simulink model "TBRe18_ECU_V7_AI"  (R2017b)
settings: Solver=FixedStepDiscrete  StartTime=0.0  StopTime=inf  FixedStep=0.0001  RelTol=1e-3
PostLoadFcn:
  | model_init();
libraries: simulink x16, simulink_extras x1
(part 3 of 4)

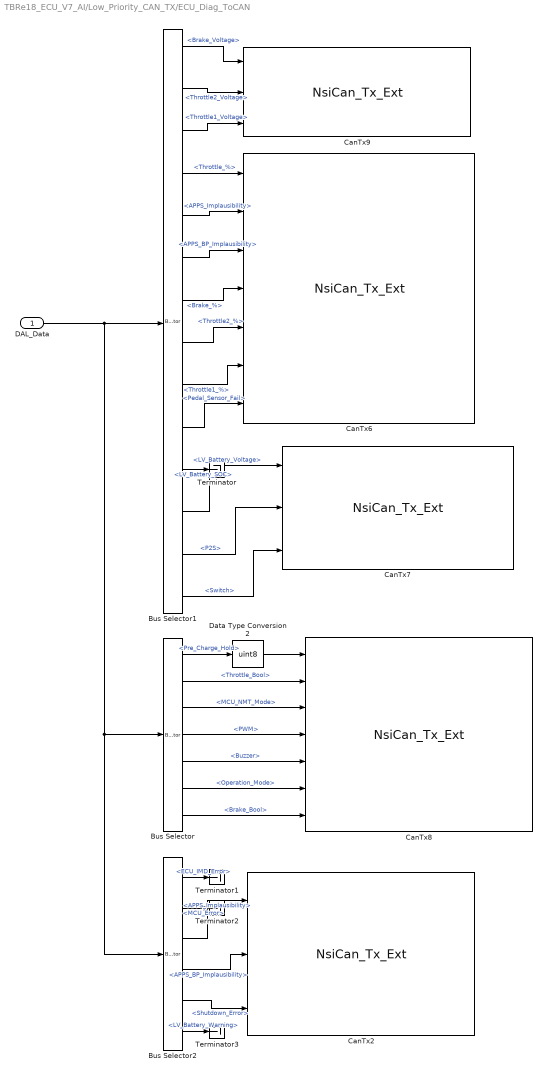
== system TBRe18_ECU_V7_AI/Low_Priority_CAN_TX/ECU_Diag_ToCAN ==
  DAL_Data : Inport
  Bus Selector : BusSelector  OutputSignals=Input_Data_Bus.BMS_Data.Pre_Charge_Hold,Vehicle_Operation_Data.Throttle_Bool,Vehicle_Operation_Data.MCU_NMT_Mode,Vehicle_Operation_Data.PWM,Vehicle_Operation_Data.Buzzer,Vehicle_Operation_Data.Operation_Mode,Vehicle_Operation_Data.Brake_Bool
  Bus Selector1 : BusSelector  OutputSignals=Input_Data_Bus.ECU_IO_Data.Pedal_Box_Data.Brake_Voltage,Input_Data_Bus.ECU_IO_Data.Pedal_Box_Data.Throttle2_Voltage,Input_Data_Bus.ECU_IO_Data.Pedal_Box_Data.Throttle1_Voltage,Input_Data_Bus.ECU_IO_Data.Pedal_Box_Data.Throttle_%,Input_Data_Bus.ECU_IO_Data.Pedal_Box_Data.APPS_Implausibility,Input_Data_Bus.ECU_IO_Data.Pedal_Box_Data.APPS_BP_Implausibility,Input_Data_Bus.ECU_IO_Data.Pedal_Box_Data.Brake_%,Input_Data_Bus.ECU_IO_Data.Pedal_Box_Data.Throttle2_%,Input_Data_Bus.ECU_IO_Data.Pedal_Box_Data.Throttle1_%,Input_Data_Bus.ECU_IO_Data.Pedal_Box_Data.Pedal_Sensor_Fail,Input_Data_Bus.ECU_IO_Data.LV_Battery_Data.LV_Battery_SOC,Input_Data_Bus.ECU_IO_Data.LV_Battery_Data.LV_Battery_Voltage,Input_Data_Bus.Console_Data.P2S,Input_Data_Bus.Console_Data.Switch
  Bus Selector2 : BusSelector  OutputSignals=Input_Data_Bus.ECU_IO_Data.IMD_Data.ECU_IMD_Error,Input_Data_Bus.MCU_Data.MCU_Error,Input_Data_Bus.ECU_IO_Data.Pedal_Box_Data.APPS_Implausibility,Input_Data_Bus.ECU_IO_Data.Pedal_Box_Data.APPS_BP_Implausibility,Input_Data_Bus.Shutdown_Data.Shutdown_Error,Input_Data_Bus.ECU_IO_Data.LV_Battery_Data.LV_Battery_Warning
  CanTx2 : S-Function  FunctionName=NsiCan_Tx_Ext  Parameters=data_can,channel,msg_name,ident,ident_type,dlc,signals,is_physical,is_canfd,is_crc  SFunctionDeploymentMode=off  EnableBusSupport=off  mask(MUXlink Can Tx){data_can=1;HIGH_SPEED;500Kbps;120 Ohm;C:\Users\TBRe-admin\Documents\MATLAB\TBRe18_DBC_190304.dbc;0;;;1;LOW_SPEED;125Kbps;560 Ohm;C:\Users\TBRe-admin\Documents\MATLAB\TBRe18_DBC_190304.dbc;0;;;0;HIGH_SPEED;1000Kbps;120 Ohm;D:\TOOLS\MUXLINK\R2011b\MUXlink\misc\BASE_CAN_MUXLAB4.dbc;0;;;0;HIGH_SPEED;500Kbps;120 Ohm;D:\TOOLS\MUXLINK\R2011b\MUXlink\misc\j1939_adapt.dbc;0;;;0;HIGH_SPEED;1000Kbps;No;D:\TOOLS\MUXLINK\R2011b\MUXlink\misc\BASE_CAN_MUXLAB4.dbc;0;;, channel=2, msg_name=ECU_Diagnostics, ident=0x700, ident_type=STD, dlc=4, signals=APPS_Implausibility;1;4;1;1.000000;0.000000;_;APPS_BP_Implausibility;1;3;1;1.000000;0.000000;_;Shutdown_Error;1;2;1;1.000000;0.000000;_, is_physical=0, is_canfd=0, is_crc=0}
      mask prompts: data_can "data can"; msg_name "msg name"
      mask help: Transmit a frame on a CAN Channel.
      mask init:
      | NsiCan_Tx_Ext_InitializationFcn();
      settings: OpenFcn=NsiCan_Tx_Ext_OpenFcn();
      mask Help:
      | eval('block=get_param(gcb, ''RTWdata'');')
      | web([docroot '\toolbox\MUXlink\html\blocks/' block.MUXlink_BlockType '.html'])
      mask Callback data_can: NsiCan_Tx_Ext_ApplyFcn(1);
      mask Callback channel: NsiCan_Tx_Ext_ApplyFcn(2);
      mask Callback msg_name: NsiCan_Tx_Ext_ApplyFcn(3);
      mask Callback ident: NsiCan_Tx_Ext_ApplyFcn(4);
      mask Callback ident_type: NsiCan_Tx_Ext_ApplyFcn(5);
      mask Callback dlc: NsiCan_Tx_Ext_ApplyFcn(6);
      mask Callback signals: NsiCan_Tx_Ext_ApplyFcn(7);
      mask Callback is_physical: NsiCan_Tx_Ext_ApplyFcn(7);
      mask Callback is_canfd: NsiCan_Tx_Ext_ApplyFcn(7);
      mask Callback is_crc: NsiCan_Tx_Ext_ApplyFcn(7);
      mask Display: image(imread('nsi.bmp'));text(0.5, 0.1, 'TX_ECU_Diagnostics_CAN2', 'horizontalAlignment', 'center', 'verticalAlignment', 'base');plot([0.05 0.05 0.05 0.05 0.05 0.05 0.05 0.05 0.05 0.05]); port_label('input',1, 'APPS_Implausibility'); port_label('input',2, 'APPS_BP_Implausibility'); port_label('input',3, 'Shutdown_Error');
  CanTx6 : S-Function  FunctionName=NsiCan_Tx_Ext  Parameters=data_can,channel,msg_name,ident,ident_type,dlc,signals,is_physical,is_canfd,is_crc  SFunctionDeploymentMode=off  EnableBusSupport=off  mask(MUXlink Can Tx){data_can=1;HIGH_SPEED;500Kbps;120 Ohm;C:\Users\TBRe-admin\Documents\MATLAB\TBRe18_DBC_190304.dbc;0;;;1;LOW_SPEED;125Kbps;560 Ohm;C:\Users\TBRe-admin\Documents\MATLAB\TBRe18_DBC_190304.dbc;0;;;0;HIGH_SPEED;1000Kbps;120 Ohm;D:\TOOLS\MUXLINK\R2011b\MUXlink\misc\BASE_CAN_MUXLAB4.dbc;0;;;0;HIGH_SPEED;500Kbps;120 Ohm;D:\TOOLS\MUXLINK\R2011b\MUXlink\misc\j1939_adapt.dbc;0;;;0;HIGH_SPEED;1000Kbps;No;D:\TOOLS\MUXLINK\R2011b\MUXlink\misc\BASE_CAN_MUXLAB4.dbc;0;;, channel=2, msg_name=ECU_Pedal_Box_Data, ident=0x702, ident_type=STD, dlc=5, signals=Throttle_Percentage;1;32;8;1.000000;0.000000;_;APPS_Implausibility;1;4;1;1.000000;0.000000;_;APPS_BP_Implausibility;1;3;1;1.000000;0.000000;_;Brake_Percentage;1;24;8;1.000000;0.000000;_;Throttle2_Percentage;1;16;8;1.000000;0.000000;_;Throttle1_Percent;1;8;8;1.000000;0.000000;_;Pedal_Sensor_Fail;1;0;3;1.000000;0.000000;_, is_physical=0, is_canfd=0, is_crc=0}
      mask prompts: data_can "data can"; msg_name "msg name"
      mask help: Transmit a frame on a CAN Channel.
      mask init:
      | NsiCan_Tx_Ext_InitializationFcn();
      settings: OpenFcn=NsiCan_Tx_Ext_OpenFcn();
      mask Help:
      | eval('block=get_param(gcb, ''RTWdata'');')
      | web([docroot '\toolbox\MUXlink\html\blocks/' block.MUXlink_BlockType '.html'])
      mask Callback data_can: NsiCan_Tx_Ext_ApplyFcn(1);
      mask Callback channel: NsiCan_Tx_Ext_ApplyFcn(2);
      mask Callback msg_name: NsiCan_Tx_Ext_ApplyFcn(3);
      mask Callback ident: NsiCan_Tx_Ext_ApplyFcn(4);
      mask Callback ident_type: NsiCan_Tx_Ext_ApplyFcn(5);
      mask Callback dlc: NsiCan_Tx_Ext_ApplyFcn(6);
      mask Callback signals: NsiCan_Tx_Ext_ApplyFcn(7);
      mask Callback is_physical: NsiCan_Tx_Ext_ApplyFcn(7);
      mask Callback is_canfd: NsiCan_Tx_Ext_ApplyFcn(7);
      mask Callback is_crc: NsiCan_Tx_Ext_ApplyFcn(7);
      mask Display: image(imread('nsi.bmp'));text(0.5, 0.1, 'TX_ECU_Pedal_Box_Data_CAN2', 'horizontalAlignment', 'center', 'verticalAlignment', 'base');plot([0.05 0.05 0.05 0.05 0.05 0.05 0.05 0.05 0.05 0.05]); port_label('input',1, 'Throttle_Percentage'); port_label('input',2, 'APPS_Implausibility'); port_label('input',3, 'APPS_BP_Implausibility'); port_label('input',4, 'Brake_Percentage'); port_label('input',5, 'Throttle2_Percentage'); port_label('input',6, 'Throttle1_Percent'); port_label('input',7, 'Pedal_Sensor_Fail');
  CanTx7 : S-Function  FunctionName=NsiCan_Tx_Ext  Parameters=data_can,channel,msg_name,ident,ident_type,dlc,signals,is_physical,is_canfd,is_crc  SFunctionDeploymentMode=off  EnableBusSupport=off  mask(MUXlink Can Tx){data_can=1;HIGH_SPEED;500Kbps;120 Ohm;C:\Users\TBRe-admin\Documents\MATLAB\TBRe18_DBC_190304.dbc;0;;;1;LOW_SPEED;125Kbps;560 Ohm;C:\Users\TBRe-admin\Documents\MATLAB\TBRe18_DBC_190304.dbc;0;;;0;HIGH_SPEED;1000Kbps;120 Ohm;D:\TOOLS\MUXLINK\R2011b\MUXlink\misc\BASE_CAN_MUXLAB4.dbc;0;;;0;HIGH_SPEED;500Kbps;120 Ohm;D:\TOOLS\MUXLINK\R2011b\MUXlink\misc\j1939_adapt.dbc;0;;;0;HIGH_SPEED;1000Kbps;No;D:\TOOLS\MUXLINK\R2011b\MUXlink\misc\BASE_CAN_MUXLAB4.dbc;0;;, channel=2, msg_name=ECU_HW_IO, ident=0x701, ident_type=STD, dlc=4, signals=LV_Battery_Voltage;1;16;16;1.000000;0.000000;mV;Console_Push_to_Start;1;9;1;1.000000;0.000000;Bool;Console_Reset;1;8;1;1.000000;0.000000;Bool, is_physical=0, is_canfd=0, is_crc=0}
      mask prompts: data_can "data can"; msg_name "msg name"
      mask help: Transmit a frame on a CAN Channel.
      mask init:
      | NsiCan_Tx_Ext_InitializationFcn();
      settings: OpenFcn=NsiCan_Tx_Ext_OpenFcn();
      mask Help:
      | eval('block=get_param(gcb, ''RTWdata'');')
      | web([docroot '\toolbox\MUXlink\html\blocks/' block.MUXlink_BlockType '.html'])
      mask Callback data_can: NsiCan_Tx_Ext_ApplyFcn(1);
      mask Callback channel: NsiCan_Tx_Ext_ApplyFcn(2);
      mask Callback msg_name: NsiCan_Tx_Ext_ApplyFcn(3);
      mask Callback ident: NsiCan_Tx_Ext_ApplyFcn(4);
      mask Callback ident_type: NsiCan_Tx_Ext_ApplyFcn(5);
      mask Callback dlc: NsiCan_Tx_Ext_ApplyFcn(6);
      mask Callback signals: NsiCan_Tx_Ext_ApplyFcn(7);
      mask Callback is_physical: NsiCan_Tx_Ext_ApplyFcn(7);
      mask Callback is_canfd: NsiCan_Tx_Ext_ApplyFcn(7);
      mask Callback is_crc: NsiCan_Tx_Ext_ApplyFcn(7);
      mask Display: image(imread('nsi.bmp'));text(0.5, 0.1, 'TX_ECU_HW_IO_CAN2', 'horizontalAlignment', 'center', 'verticalAlignment', 'base');plot([0.05 0.05 0.05 0.05 0.05 0.05 0.05 0.05 0.05 0.05]); port_label('input',1, 'LV_Battery_Voltage'); port_label('input',2, 'Console_Push_to_Start'); port_label('input',3, 'Console_Reset');
  CanTx8 : S-Function  FunctionName=NsiCan_Tx_Ext  Parameters=data_can,channel,msg_name,ident,ident_type,dlc,signals,is_physical,is_canfd,is_crc  SFunctionDeploymentMode=off  EnableBusSupport=off  mask(MUXlink Can Tx){data_can=1;HIGH_SPEED;500Kbps;120 Ohm;C:\Users\TBRe-admin\Documents\MATLAB\TBRe18_DBC_190304.dbc;0;;;1;LOW_SPEED;125Kbps;560 Ohm;C:\Users\TBRe-admin\Documents\MATLAB\TBRe18_DBC_190304.dbc;0;;;0;HIGH_SPEED;1000Kbps;120 Ohm;D:\TOOLS\MUXLINK\R2011b\MUXlink\misc\BASE_CAN_MUXLAB4.dbc;0;;;0;HIGH_SPEED;500Kbps;120 Ohm;D:\TOOLS\MUXLINK\R2011b\MUXlink\misc\j1939_adapt.dbc;0;;;0;HIGH_SPEED;1000Kbps;No;D:\TOOLS\MUXLINK\R2011b\MUXlink\misc\BASE_CAN_MUXLAB4.dbc;0;;, channel=2, msg_name=ECU_Vehicle_Functionality, ident=0x704, ident_type=STD, dlc=4, signals=Pre_Charge;1;24;8;1.000000;0.000000;_;Throttle_Bool;1;2;1;1.000000;0.000000;_;MCU_NMT_Mode;1;16;8;1.000000;0.000000;_;PWM;1;3;1;1.000000;0.000000;_;Buzzer;1;1;1;1.000000;0.000000;_;Vehicle_Operation;1;8;8;1.000000;0.000000;_;Brake_Bool;1;0;1;1.000000;0.000000;_, is_physical=0, is_canfd=0, is_crc=0}
      mask prompts: data_can "data can"; msg_name "msg name"
      mask help: Transmit a frame on a CAN Channel.
      mask init:
      | NsiCan_Tx_Ext_InitializationFcn();
      settings: OpenFcn=NsiCan_Tx_Ext_OpenFcn();
      mask Help:
      | eval('block=get_param(gcb, ''RTWdata'');')
      | web([docroot '\toolbox\MUXlink\html\blocks/' block.MUXlink_BlockType '.html'])
      mask Callback data_can: NsiCan_Tx_Ext_ApplyFcn(1);
      mask Callback channel: NsiCan_Tx_Ext_ApplyFcn(2);
      mask Callback msg_name: NsiCan_Tx_Ext_ApplyFcn(3);
      mask Callback ident: NsiCan_Tx_Ext_ApplyFcn(4);
      mask Callback ident_type: NsiCan_Tx_Ext_ApplyFcn(5);
      mask Callback dlc: NsiCan_Tx_Ext_ApplyFcn(6);
      mask Callback signals: NsiCan_Tx_Ext_ApplyFcn(7);
      mask Callback is_physical: NsiCan_Tx_Ext_ApplyFcn(7);
      mask Callback is_canfd: NsiCan_Tx_Ext_ApplyFcn(7);
      mask Callback is_crc: NsiCan_Tx_Ext_ApplyFcn(7);
      mask Display: image(imread('nsi.bmp'));text(0.5, 0.1, 'TX_ECU_Vehicle_Functionality_CAN2', 'horizontalAlignment', 'center', 'verticalAlignment', 'base');plot([0.05 0.05 0.05 0.05 0.05 0.05 0.05 0.05 0.05 0.05]); port_label('input',1, 'Pre_Charge'); port_label('input',2, 'Throttle_Bool'); port_label('input',3, 'MCU_NMT_Mode'); port_label('input',4, 'PWM'); port_label('input',5, 'Buzzer'); port_label('input',6, 'Vehicle_Operation'); port_label('input',7, 'Brake_Bool');
  CanTx9 : S-Function  FunctionName=NsiCan_Tx_Ext  Parameters=data_can,channel,msg_name,ident,ident_type,dlc,signals,is_physical,is_canfd,is_crc  SFunctionDeploymentMode=off  EnableBusSupport=off  mask(MUXlink Can Tx){data_can=1;HIGH_SPEED;500Kbps;120 Ohm;C:\Users\TBRe-admin\Documents\MATLAB\TBRe18_DBC_190304.dbc;0;;;1;LOW_SPEED;125Kbps;560 Ohm;C:\Users\TBRe-admin\Documents\MATLAB\TBRe18_DBC_190304.dbc;0;;;0;HIGH_SPEED;1000Kbps;120 Ohm;D:\TOOLS\MUXLINK\R2011b\MUXlink\misc\BASE_CAN_MUXLAB4.dbc;0;;;0;HIGH_SPEED;500Kbps;120 Ohm;D:\TOOLS\MUXLINK\R2011b\MUXlink\misc\j1939_adapt.dbc;0;;;0;HIGH_SPEED;1000Kbps;No;D:\TOOLS\MUXLINK\R2011b\MUXlink\misc\BASE_CAN_MUXLAB4.dbc;0;;, channel=2, msg_name=ECU_Pedal_Voltages, ident=0x703, ident_type=STD, dlc=8, signals=Brake_Voltage;1;32;16;1.000000;0.000000;mV;Throttle2_Voltage;1;48;16;1.000000;0.000000;_;Throttle1_Voltage;1;0;16;1.000000;0.000000;_, is_physical=0, is_canfd=0, is_crc=0}
      mask prompts: data_can "data can"; msg_name "msg name"
      mask help: Transmit a frame on a CAN Channel.
      mask init:
      | NsiCan_Tx_Ext_InitializationFcn();
      settings: OpenFcn=NsiCan_Tx_Ext_OpenFcn();
      mask Help:
      | eval('block=get_param(gcb, ''RTWdata'');')
      | web([docroot '\toolbox\MUXlink\html\blocks/' block.MUXlink_BlockType '.html'])
      mask Callback data_can: NsiCan_Tx_Ext_ApplyFcn(1);
      mask Callback channel: NsiCan_Tx_Ext_ApplyFcn(2);
      mask Callback msg_name: NsiCan_Tx_Ext_ApplyFcn(3);
      mask Callback ident: NsiCan_Tx_Ext_ApplyFcn(4);
      mask Callback ident_type: NsiCan_Tx_Ext_ApplyFcn(5);
      mask Callback dlc: NsiCan_Tx_Ext_ApplyFcn(6);
      mask Callback signals: NsiCan_Tx_Ext_ApplyFcn(7);
      mask Callback is_physical: NsiCan_Tx_Ext_ApplyFcn(7);
      mask Callback is_canfd: NsiCan_Tx_Ext_ApplyFcn(7);
      mask Callback is_crc: NsiCan_Tx_Ext_ApplyFcn(7);
      mask Display: image(imread('nsi.bmp'));text(0.5, 0.1, 'TX_ECU_Pedal_Voltages_CAN2', 'horizontalAlignment', 'center', 'verticalAlignment', 'base');plot([0.05 0.05 0.05 0.05 0.05 0.05 0.05 0.05 0.05 0.05]); port_label('input',1, 'Brake_Voltage'); port_label('input',2, 'Throttle2_Voltage'); port_label('input',3, 'Throttle1_Voltage');
  Data Type Conversion2 : DataTypeConversion  OutDataTypeStr=uint8
  Terminator{,1..3} (4 alike) : Terminator
  wires:
  Bus Selector1/4 -> CanTx6/1  "<Throttle_%>"
  Bus Selector1/5 -> CanTx6/2  "<APPS_Implausibility>"
  Bus Selector1/6 -> CanTx6/3  "<APPS_BP_Implausibility>"
  Bus Selector1/7 -> CanTx6/4  "<Brake_%>"
  Bus Selector1/8 -> CanTx6/5  "<Throttle2_%>"
  Bus Selector1/9 -> CanTx6/6  "<Throttle1_%>"
  Bus Selector1/10 -> CanTx6/7  "<Pedal_Sensor_Fail>"
  Bus Selector1/1 -> CanTx9/1  "<Brake_Voltage>"
  Bus Selector1/2 -> CanTx9/2  "<Throttle2_Voltage>"
  Bus Selector1/3 -> CanTx9/3  "<Throttle1_Voltage>"
  Bus Selector/7 -> CanTx8/7  "<Brake_Bool>"
  Bus Selector2/4 -> CanTx2/2  "<APPS_BP_Implausibility>"
  Bus Selector1/13 -> CanTx7/2  "<P2S>"
  Bus Selector/2 -> CanTx8/2  "<Throttle_Bool>"
  Bus Selector/3 -> CanTx8/3  "<MCU_NMT_Mode>"
  Bus Selector/4 -> CanTx8/4  "<PWM>"
  Bus Selector/6 -> CanTx8/6  "<Operation_Mode>"
  Bus Selector/5 -> CanTx8/5  "<Buzzer>"
  DAL_Data/1 -> Bus Selector1/1, Bus Selector/1, Bus Selector2/1
  Bus Selector2/5 -> CanTx2/3  "<Shutdown_Error>"
  Bus Selector2/3 -> CanTx2/1  "<APPS_Implausibility>"
  Data Type Conversion2/1 -> CanTx8/1
  Bus Selector/1 -> Data Type Conversion2/1  "<Pre_Charge_Hold>"
  Bus Selector1/12 -> CanTx7/1  "<LV_Battery_Voltage>"
  Bus Selector1/14 -> CanTx7/3  "<Switch>"
  Bus Selector1/11 -> Terminator/1  "<LV_Battery_SOC>"
  Bus Selector2/1 -> Terminator1/1  "<ECU_IMD_Error>"
  Bus Selector2/2 -> Terminator2/1  "<MCU_Error>"
  Bus Selector2/6 -> Terminator3/1  "<LV_Battery_Warning>"

== system TBRe18_ECU_V7_AI/Low_Priority_CAN_TX/Init ==

== system TBRe18_ECU_V7_AI/Low_Priority_CAN_TX/MCU_Diag_ToCAN ==
  DAL_Data : Inport
  Bus Selector : BusSelector  OutputSignals=Input_Data_Bus.MCU_Data.DC_Link_Current,Input_Data_Bus.MCU_Data.DC_Link_Voltage,Input_Data_Bus.MCU_Data.Motor_Temp,Input_Data_Bus.MCU_Data.MCU_Temp
  CanRx1 : S-Function  FunctionName=NsiCan_Rx_Ext  Parameters=data_can,channel,msg_name,ident,ident_type,dlc,signals,is_trigger,is_physical,is_canfd,is_rxgw  SFunctionDeploymentMode=off  EnableBusSupport=off  mask(MUXlink Can Rx){data_can=1;HIGH_SPEED;500Kbps;120 Ohm;C:\Users\TBRe-admin\Documents\MATLAB\TBRe18_DBC_190304.dbc;0;;;1;LOW_SPEED;125Kbps;560 Ohm;C:\Users\TBRe-admin\Documents\MATLAB\TBRe18_DBC_190304.dbc;0;;;0;HIGH_SPEED;1000Kbps;120 Ohm;D:\TOOLS\MUXLINK\R2011b\MUXlink\misc\BASE_CAN_MUXLAB4.dbc;0;;;0;HIGH_SPEED;500Kbps;120 Ohm;D:\TOOLS\MUXLINK\R2011b\MUXlink\misc\j1939_adapt.dbc;0;;;0;HIGH_SPEED;1000Kbps;No;D:\TOOLS\MUXLINK\R2011b\MUXlink\misc\BASE_CAN_MUXLAB4.dbc;0;;, channel=1, msg_name=MCU_TPDO3, ident=0x381, ident_type=STD, dlc=8, signals=MCU_Error_Code;1;0;-16;1.000000;0.000000;_;MCU_Status_Word;1;16;16;1.000000;0.000000;_;MCU_PhaseB_Current;1;48;-16;1.000000;0.000000;_;MCU_PhaseA_Current;1;32;-16;1.000000;0.000000;_, is_trigger=0, is_physical=0, is_canfd=0, is_rxgw=0}
      mask prompts: data_can "data can"; msg_name "msg name"
      mask help: Receive a frame from a CAN channel.
      mask init:
      | NsiCan_Rx_Ext_InitializationFcn();
      settings: OpenFcn=NsiCan_Rx_Ext_OpenFcn();
      mask Help:
      | eval('block=get_param(gcb, ''RTWdata'');')
      | web([docroot '\toolbox\MUXlink\html\blocks/' block.MUXlink_BlockType '.html'])
      mask Callback data_can: NsiCan_Rx_Ext_ApplyFcn(1);
      mask Callback channel: NsiCan_Rx_Ext_ApplyFcn(2);
      mask Callback msg_name: NsiCan_Rx_Ext_ApplyFcn(3);
      mask Callback ident: NsiCan_Rx_Ext_ApplyFcn(4);
      mask Callback ident_type: NsiCan_Rx_Ext_ApplyFcn(5);
      mask Callback dlc: NsiCan_Rx_Ext_ApplyFcn(6);
      mask Callback signals: NsiCan_Rx_Ext_ApplyFcn(7);
      mask Callback is_trigger: NsiCan_Rx_Ext_ApplyFcn(8);
      mask Callback is_physical: NsiCan_Rx_Ext_ApplyFcn(9);
      mask Callback is_canfd: NsiCan_Rx_Ext_ApplyFcn(10);
      mask Callback is_rxgw: NsiCan_Rx_Ext_ApplyFcn(11);
      mask Display: image(imread('nsi.bmp'));text(0.5, 0.3, 'RX_MCU_TPDO3_CAN1', 'horizontalAlignment', 'center', 'verticalAlignment', 'base');plot([0.05 0.05 0.05 0.05 0.05 0.05 0.05 0.05 0.05 0.05]); port_label('output',1, 'MCU_Error_Code'); port_label('output',2, 'MCU_Status_Word'); port_label('output',3, 'MCU_PhaseB_Current'); port_label('output',4, 'MCU_PhaseA_Current'); port_label('output',5, 'Status');
  CanRx2 : S-Function  FunctionName=NsiCan_Rx_Ext  Parameters=data_can,channel,msg_name,ident,ident_type,dlc,signals,is_trigger,is_physical,is_canfd,is_rxgw  SFunctionDeploymentMode=off  EnableBusSupport=off  mask(MUXlink Can Rx){data_can=1;HIGH_SPEED;500Kbps;120 Ohm;C:\Users\TBRe-admin\Documents\MATLAB\TBRe18_DBC_190304.dbc;0;;;1;LOW_SPEED;125Kbps;560 Ohm;C:\Users\TBRe-admin\Documents\MATLAB\TBRe18_DBC_190304.dbc;0;;;0;HIGH_SPEED;1000Kbps;120 Ohm;D:\TOOLS\MUXLINK\R2011b\MUXlink\misc\BASE_CAN_MUXLAB4.dbc;0;;;0;HIGH_SPEED;500Kbps;120 Ohm;D:\TOOLS\MUXLINK\R2011b\MUXlink\misc\j1939_adapt.dbc;0;;;0;HIGH_SPEED;1000Kbps;No;D:\TOOLS\MUXLINK\R2011b\MUXlink\misc\BASE_CAN_MUXLAB4.dbc;0;;, channel=1, msg_name=MCU_TPDO4, ident=0x481, ident_type=STD, dlc=8, signals=MCU_DC_Power;1;0;-32;1.000000;0.000000;W;MCU_Velocity_Actual_Value;1;32;-32;1.000000;0.000000;_, is_trigger=0, is_physical=0, is_canfd=0, is_rxgw=0}
      mask prompts: data_can "data can"; msg_name "msg name"
      mask help: Receive a frame from a CAN channel.
      mask init:
      | NsiCan_Rx_Ext_InitializationFcn();
      settings: OpenFcn=NsiCan_Rx_Ext_OpenFcn();
      mask Help:
      | eval('block=get_param(gcb, ''RTWdata'');')
      | web([docroot '\toolbox\MUXlink\html\blocks/' block.MUXlink_BlockType '.html'])
      mask Callback data_can: NsiCan_Rx_Ext_ApplyFcn(1);
      mask Callback channel: NsiCan_Rx_Ext_ApplyFcn(2);
      mask Callback msg_name: NsiCan_Rx_Ext_ApplyFcn(3);
      mask Callback ident: NsiCan_Rx_Ext_ApplyFcn(4);
      mask Callback ident_type: NsiCan_Rx_Ext_ApplyFcn(5);
      mask Callback dlc: NsiCan_Rx_Ext_ApplyFcn(6);
      mask Callback signals: NsiCan_Rx_Ext_ApplyFcn(7);
      mask Callback is_trigger: NsiCan_Rx_Ext_ApplyFcn(8);
      mask Callback is_physical: NsiCan_Rx_Ext_ApplyFcn(9);
      mask Callback is_canfd: NsiCan_Rx_Ext_ApplyFcn(10);
      mask Callback is_rxgw: NsiCan_Rx_Ext_ApplyFcn(11);
      mask Display: image(imread('nsi.bmp'));text(0.5, 0.3, 'RX_MCU_TPDO4_CAN1', 'horizontalAlignment', 'center', 'verticalAlignment', 'base');plot([0.05 0.05 0.05 0.05 0.05 0.05 0.05 0.05 0.05 0.05]); port_label('output',1, 'MCU_DC_Power'); port_label('output',2, 'MCU_Velocity_Actual_Value'); port_label('output',3, 'Status');
  CanTx2 : S-Function  FunctionName=NsiCan_Tx_Ext  Parameters=data_can,channel,msg_name,ident,ident_type,dlc,signals,is_physical,is_canfd,is_crc  SFunctionDeploymentMode=off  EnableBusSupport=off  mask(MUXlink Can Tx){data_can=1;HIGH_SPEED;500Kbps;120 Ohm;C:\Users\TBRe-admin\Documents\MATLAB\TBRe18_DBC_190304.dbc;0;;;1;LOW_SPEED;125Kbps;560 Ohm;C:\Users\TBRe-admin\Documents\MATLAB\TBRe18_DBC_190304.dbc;0;;;0;HIGH_SPEED;1000Kbps;120 Ohm;D:\TOOLS\MUXLINK\R2011b\MUXlink\misc\BASE_CAN_MUXLAB4.dbc;0;;;0;HIGH_SPEED;500Kbps;120 Ohm;D:\TOOLS\MUXLINK\R2011b\MUXlink\misc\j1939_adapt.dbc;0;;;0;HIGH_SPEED;1000Kbps;No;D:\TOOLS\MUXLINK\R2011b\MUXlink\misc\BASE_CAN_MUXLAB4.dbc;0;;, channel=1, msg_name=MCU_TPDO4, ident=0x481, ident_type=STD, dlc=8, signals=MCU_DC_Power;1;0;-32;1.000000;0.000000;W;MCU_Velocity_Actual_Value;1;32;-32;1.000000;0.000000;_, is_physical=0, is_canfd=0, is_crc=0}
      mask prompts: data_can "data can"; msg_name "msg name"
      mask help: Transmit a frame on a CAN Channel.
      mask init:
      | NsiCan_Tx_Ext_InitializationFcn();
      settings: OpenFcn=NsiCan_Tx_Ext_OpenFcn();
      mask Help:
      | eval('block=get_param(gcb, ''RTWdata'');')
      | web([docroot '\toolbox\MUXlink\html\blocks/' block.MUXlink_BlockType '.html'])
      mask Callback data_can: NsiCan_Tx_Ext_ApplyFcn(1);
      mask Callback channel: NsiCan_Tx_Ext_ApplyFcn(2);
      mask Callback msg_name: NsiCan_Tx_Ext_ApplyFcn(3);
      mask Callback ident: NsiCan_Tx_Ext_ApplyFcn(4);
      mask Callback ident_type: NsiCan_Tx_Ext_ApplyFcn(5);
      mask Callback dlc: NsiCan_Tx_Ext_ApplyFcn(6);
      mask Callback signals: NsiCan_Tx_Ext_ApplyFcn(7);
      mask Callback is_physical: NsiCan_Tx_Ext_ApplyFcn(7);
      mask Callback is_canfd: NsiCan_Tx_Ext_ApplyFcn(7);
      mask Callback is_crc: NsiCan_Tx_Ext_ApplyFcn(7);
      mask Display: image(imread('nsi.bmp'));text(0.5, 0.3, 'TX_MCU_TPDO4_CAN1', 'horizontalAlignment', 'center', 'verticalAlignment', 'base');plot([0.05 0.05 0.05 0.05 0.05 0.05 0.05 0.05 0.05 0.05]); port_label('input',1, 'MCU_DC_Power'); port_label('input',2, 'MCU_Velocity_Actual_Value');
  CanTx3 : S-Function  FunctionName=NsiCan_Tx_Ext  Parameters=data_can,channel,msg_name,ident,ident_type,dlc,signals,is_physical,is_canfd,is_crc  SFunctionDeploymentMode=off  EnableBusSupport=off  mask(MUXlink Can Tx){data_can=1;HIGH_SPEED;500Kbps;120 Ohm;C:\Users\TBRe-admin\Documents\MATLAB\TBRe18_DBC_190304.dbc;0;;;1;LOW_SPEED;125Kbps;560 Ohm;C:\Users\TBRe-admin\Documents\MATLAB\TBRe18_DBC_190304.dbc;0;;;0;HIGH_SPEED;1000Kbps;120 Ohm;D:\TOOLS\MUXLINK\R2011b\MUXlink\misc\BASE_CAN_MUXLAB4.dbc;0;;;0;HIGH_SPEED;500Kbps;120 Ohm;D:\TOOLS\MUXLINK\R2011b\MUXlink\misc\j1939_adapt.dbc;0;;;0;HIGH_SPEED;1000Kbps;No;D:\TOOLS\MUXLINK\R2011b\MUXlink\misc\BASE_CAN_MUXLAB4.dbc;0;;, channel=2, msg_name=MCU_TPDO2, ident=0x281, ident_type=STD, dlc=8, signals=MCU_DC_Link_Current;1;32;-32;1.000000;0.000000;_;MCU_DC_Link_Voltage;1;16;-16;1.000000;0.000000;_;Motor_Temp;1;8;8;1.000000;0.000000;_;MCU_Temp;1;0;8;1.000000;0.000000;_, is_physical=0, is_canfd=0, is_crc=0}
      mask prompts: data_can "data can"; msg_name "msg name"
      mask help: Transmit a frame on a CAN Channel.
      mask init:
      | NsiCan_Tx_Ext_InitializationFcn();
      settings: OpenFcn=NsiCan_Tx_Ext_OpenFcn();
      mask Help:
      | eval('block=get_param(gcb, ''RTWdata'');')
      | web([docroot '\toolbox\MUXlink\html\blocks/' block.MUXlink_BlockType '.html'])
      mask Callback data_can: NsiCan_Tx_Ext_ApplyFcn(1);
      mask Callback channel: NsiCan_Tx_Ext_ApplyFcn(2);
      mask Callback msg_name: NsiCan_Tx_Ext_ApplyFcn(3);
      mask Callback ident: NsiCan_Tx_Ext_ApplyFcn(4);
      mask Callback ident_type: NsiCan_Tx_Ext_ApplyFcn(5);
      mask Callback dlc: NsiCan_Tx_Ext_ApplyFcn(6);
      mask Callback signals: NsiCan_Tx_Ext_ApplyFcn(7);
      mask Callback is_physical: NsiCan_Tx_Ext_ApplyFcn(7);
      mask Callback is_canfd: NsiCan_Tx_Ext_ApplyFcn(7);
      mask Callback is_crc: NsiCan_Tx_Ext_ApplyFcn(7);
      mask Display: image(imread('nsi.bmp'));text(0.5, 0.3, 'TX_MCU_TPDO2_CAN2', 'horizontalAlignment', 'center', 'verticalAlignment', 'base');plot([0.05 0.05 0.05 0.05 0.05 0.05 0.05 0.05 0.05 0.05]); port_label('input',1, 'MCU_DC_Link_Current'); port_label('input',2, 'MCU_DC_Link_Voltage'); port_label('input',3, 'Motor_Temp'); port_label('input',4, 'MCU_Temp');
  CanTx4 : S-Function  FunctionName=NsiCan_Tx_Ext  Parameters=data_can,channel,msg_name,ident,ident_type,dlc,signals,is_physical,is_canfd,is_crc  SFunctionDeploymentMode=off  EnableBusSupport=off  mask(MUXlink Can Tx){data_can=1;HIGH_SPEED;500Kbps;120 Ohm;C:\Users\TBRe-admin\Documents\MATLAB\TBRe18_DBC_190304.dbc;0;;;1;LOW_SPEED;125Kbps;560 Ohm;C:\Users\TBRe-admin\Documents\MATLAB\TBRe18_DBC_190304.dbc;0;;;0;HIGH_SPEED;1000Kbps;120 Ohm;D:\TOOLS\MUXLINK\R2011b\MUXlink\misc\BASE_CAN_MUXLAB4.dbc;0;;;0;HIGH_SPEED;500Kbps;120 Ohm;D:\TOOLS\MUXLINK\R2011b\MUXlink\misc\j1939_adapt.dbc;0;;;0;HIGH_SPEED;1000Kbps;No;D:\TOOLS\MUXLINK\R2011b\MUXlink\misc\BASE_CAN_MUXLAB4.dbc;0;;, channel=1, msg_name=MCU_TPDO3, ident=0x381, ident_type=STD, dlc=8, signals=MCU_Error_Code;1;0;-16;1.000000;0.000000;_;MCU_Status_Word;1;16;16;1.000000;0.000000;_;MCU_PhaseB_Current;1;48;-16;1.000000;0.000000;_;MCU_PhaseA_Current;1;32;-16;1.000000;0.000000;_, is_physical=0, is_canfd=0, is_crc=0}
      mask prompts: data_can "data can"; msg_name "msg name"
      mask help: Transmit a frame on a CAN Channel.
      mask init:
      | NsiCan_Tx_Ext_InitializationFcn();
      settings: OpenFcn=NsiCan_Tx_Ext_OpenFcn();
      mask Help:
      | eval('block=get_param(gcb, ''RTWdata'');')
      | web([docroot '\toolbox\MUXlink\html\blocks/' block.MUXlink_BlockType '.html'])
      mask Callback data_can: NsiCan_Tx_Ext_ApplyFcn(1);
      mask Callback channel: NsiCan_Tx_Ext_ApplyFcn(2);
      mask Callback msg_name: NsiCan_Tx_Ext_ApplyFcn(3);
      mask Callback ident: NsiCan_Tx_Ext_ApplyFcn(4);
      mask Callback ident_type: NsiCan_Tx_Ext_ApplyFcn(5);
      mask Callback dlc: NsiCan_Tx_Ext_ApplyFcn(6);
      mask Callback signals: NsiCan_Tx_Ext_ApplyFcn(7);
      mask Callback is_physical: NsiCan_Tx_Ext_ApplyFcn(7);
      mask Callback is_canfd: NsiCan_Tx_Ext_ApplyFcn(7);
      mask Callback is_crc: NsiCan_Tx_Ext_ApplyFcn(7);
      mask Display: image(imread('nsi.bmp'));text(0.5, 0.3, 'TX_MCU_TPDO3_CAN1', 'horizontalAlignment', 'center', 'verticalAlignment', 'base');plot([0.05 0.05 0.05 0.05 0.05 0.05 0.05 0.05 0.05 0.05]); port_label('input',1, 'MCU_Error_Code'); port_label('input',2, 'MCU_Status_Word'); port_label('input',3, 'MCU_PhaseB_Current'); port_label('input',4, 'MCU_PhaseA_Current');
  Data Type Conversion : DataTypeConversion  OutDataTypeStr=uint16  LockScale=on
  Data Type Conversion1 : DataTypeConversion  OutDataTypeStr=uint32
  Terminator1 : Terminator
  Terminator2 : Terminator
  wires:
  CanRx2/1 -> CanTx2/1
  CanRx2/2 -> CanTx2/2
  CanRx1/1 -> CanTx4/1
  CanRx1/2 -> CanTx4/2
  CanRx1/3 -> CanTx4/3
  CanRx1/4 -> CanTx4/4
  Bus Selector/3 -> CanTx3/3  "<Motor_Temp>"
  Bus Selector/4 -> CanTx3/4  "<MCU_Temp>"
  Bus Selector/2 -> Data Type Conversion/1  "<DC_Link_Voltage>"
  CanRx1/5 -> Terminator1/1
  DAL_Data/1 -> Bus Selector/1
  Data Type Conversion/1 -> CanTx3/2
  CanRx2/3 -> Terminator2/1
  Bus Selector/1 -> Data Type Conversion1/1  "<DC_Link_Current>"
  Data Type Conversion1/1 -> CanTx3/1

== system TBRe18_ECU_V7_AI/Data_Processing/Diagnostics/BMS_Diagnostics ==
  note: SDO data is reply from MCU DC Link Voltage read request when not in ready to drive, see HP CAN out
  In1 : Inport
  Bus Creator : BusCreator  Inputs=1
  Bus Selector : BusSelector  OutputSignals=LP_CAN_RX.BMS_Data.Instant_Pack_Voltage,HP_CAN_RX.MCU_DC_Link_Voltage,HP_CAN_RX.SDO_Data
  Compare To Constant : simulink/Logic and Bit Operations/Compare To Constant  relop===  const=3.0  OutDataTypeStr=boolean
  Data Store Read : DataStoreRead  DataStoreName=O_M
  Delay : Delay  DelayLength=10  InitialCondition=0
  MATLAB Function : MATLAB Function  TreatAsAtomicUnit=on
  Switch : Switch  Criteria=u2 > Threshold
  Out1 : Outport
  wires:
  Bus Creator/1 -> Out1/1
  In1/1 -> Bus Selector/1
  Bus Selector/1 -> MATLAB Function/1(Pack_Voltage)  "<Instant_Pack_Voltage>"
  MATLAB Function/1(Pre_Charge_Hold) -> Bus Creator/1  "Pre_Charge_Hold"
  Switch/1 -> MATLAB Function/2(MCU_Link_Voltage)
  Bus Selector/2 -> Switch/1  "<MCU_DC_Link_Voltage>"
  Bus Selector/3 -> Switch/3  "<SDO_Data>"
  Data Store Read/1 -> Compare To Constant/1
  Compare To Constant/1 -> Delay/1
  Delay/1 -> Switch/2

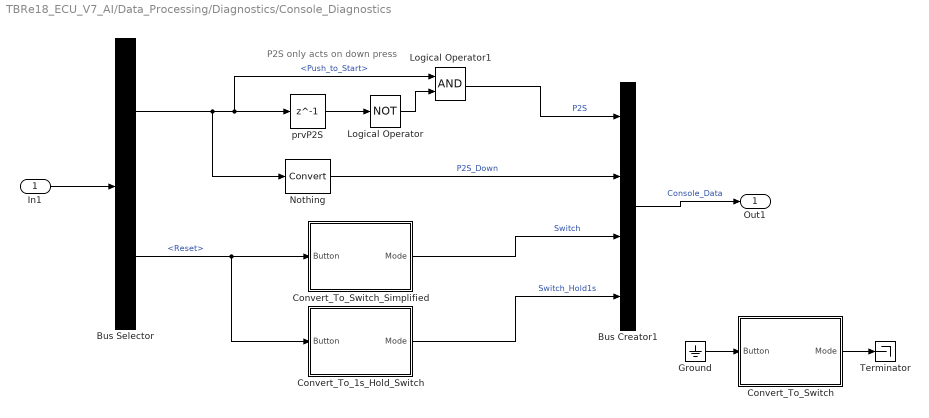
== system TBRe18_ECU_V7_AI/Data_Processing/Diagnostics/Console_Diagnostics ==
  note: P2S only acts on down press
  In1 : Inport
  Bus Creator1 : BusCreator  Inputs=4
  Bus Selector : BusSelector  OutputSignals=Hardwired_Inputs.Console_Data.Push_to_Start,Hardwired_Inputs.Console_Data.Reset
  Convert_To_1s_Hold_Switch : Subsystem  mask{initPos=false}
      mask prompts: initPos "Initial Position"
  Convert_To_Switch : Subsystem  mask{initPos=false}
      mask prompts: initPos "Initial Position"
  Convert_To_Switch_Simplified : Subsystem  mask{initPos=false}
      mask prompts: initPos "Initial Position"
  Ground : Ground
  Logical Operator : Logic  Operator=NOT  AllPortsSameDT=off  OutDataTypeStr=boolean
  Logical Operator1 : Logic  AllPortsSameDT=off  OutDataTypeStr=boolean
  Nothing : DataTypeConversion
  Terminator : Terminator
  prvP2S : Delay  DelayLength=1  InitialCondition=0
  Out1 : Outport
  wires:
  Logical Operator/1 -> Logical Operator1/2
  prvP2S/1 -> Logical Operator/1
  Logical Operator1/1 -> Bus Creator1/1  "P2S"
  Bus Creator1/1 -> Out1/1  "Console_Data"
  Bus Selector/1 -> Nothing/1, Logical Operator1/1, prvP2S/1  "<Push_to_Start>"
  Bus Selector/2 -> Convert_To_Switch_Simplified/1(Button), Convert_To_1s_Hold_Switch/1(Button)  "<Reset>"
  Convert_To_Switch_Simplified/1(Mode) -> Bus Creator1/3  "Switch"
  In1/1 -> Bus Selector/1
  Nothing/1 -> Bus Creator1/2  "P2S_Down"
  Convert_To_1s_Hold_Switch/1(Mode) -> Bus Creator1/4  "Switch_Hold1s"
  Ground/1 -> Convert_To_Switch/1(Button)
  Convert_To_Switch/1(Mode) -> Terminator/1

== system TBRe18_ECU_V7_AI/Data_Processing/Diagnostics/ECU_I//0s_Diagnostics ==
  In1 : Inport
  AIR : Subsystem
  Bus Creator : BusCreator  Inputs=4
  Bus Selector : BusSelector  OutputSignals=Hardwired_Inputs
  IMD : Subsystem
  LV_Battery : Subsystem
  Pedal_Box : Subsystem
  Out1 : Outport
  wires:
  In1/1 -> Bus Selector/1
  Bus Selector/1 -> IMD/1(In1), AIR/1(In1), LV_Battery/1(In1), Pedal_Box/1(In1)  "<Hardwired_Inputs>"
  Pedal_Box/1(Out1) -> Bus Creator/1  "Pedal_Box_Data"
  LV_Battery/1(Out1) -> Bus Creator/2  "LV_Battery_Data"
  IMD/1(Out1) -> Bus Creator/3  "IMD_Data"
  AIR/1(Out1) -> Bus Creator/4  "AIR_Data"
  Bus Creator/1 -> Out1/1

== system TBRe18_ECU_V7_AI/Data_Processing/Diagnostics/MCU_Diagnostics ==
  In1 : Inport
  Bus Creator : BusCreator  Inputs=15
  Bus Selector : BusSelector  OutputSignals=HP_CAN_RX.Motor_Temp,HP_CAN_RX.MCU_Temp
  Bus Selector1 : BusSelector  OutputSignals=HP_CAN_RX.OD_Index,HP_CAN_RX.OD_Sub_Index,HP_CAN_RX.SDO_Data
  Configuration_Check : Subsystem  Commented=on
  Error_Check : simulink/Logic and Bit Operations/Compare To Zero  Commented=on  relop=~=  OutDataTypeStr=boolean
  MCU_Error : Logic  Commented=on  Operator=OR  AllPortsSameDT=off  OutDataTypeStr=boolean
  Power Monitoring : Subsystem  Commented=on
  Temp_Check : Subsystem
  Out1 : Outport
  wires:
  Bus Creator/1 -> Out1/1
  Error_Check/1 -> MCU_Error/1
  Temp_Check/1(MCU_Temperature) -> Bus Creator/7  "MCU_Temp"
  Temp_Check/2(Motor_Temperature) -> Bus Creator/8  "Motor_Temp"
  Temp_Check/3(MCU_Motor_Temp_Error) -> Bus Creator/9  "MCU_Motor_Temp_Error"
  Temp_Check/4(MCU_Pump_Req) -> Bus Creator/10  "MCU_Pump_Req"
  MCU_Error/1 -> Bus Creator/11  "MCU_Error"
  In1/1 -> Bus Selector/1, Bus Selector1/1
  Power Monitoring/1(MCU_Power) -> Bus Creator/12  "MCU_Power"
  Power Monitoring/2(DC_Link_Voltage) -> Bus Creator/13  "DC_Link_Voltage"
  Power Monitoring/3(DC_Link_Current) -> Bus Creator/14  "DC_Link_Current"
  Power Monitoring/4(Power_Limit_Breach) -> Bus Creator/15  "Power_Limit_Breach"
  Bus Selector1/1 -> Configuration_Check/1(OD_Index_In)  "<OD_Index>"
  Bus Selector1/2 -> Configuration_Check/2(OD_Sub_Index_In)  "<OD_Sub_Index>"
  Bus Selector1/3 -> Configuration_Check/3(SDO_Data_In)  "<SDO_Data>"
  Configuration_Check/1(SDO_Specifier) -> Bus Creator/1  "SDO_Specifier"
  Configuration_Check/2(OD_Index_Out) -> Bus Creator/2  "OD_Index_Out"
  Configuration_Check/3(OD_Sub_Index_Out) -> Bus Creator/3  "OD_Sub_Index"
  Configuration_Check/4(SDO_Data_Out) -> Bus Creator/4  "SDO_Data_Out"
  Configuration_Check/5(MCU_Config_Error) -> Bus Creator/5  "MCU_Config_Error"
  Bus Selector/1 -> Temp_Check/1(MCU_Temp)  "<Motor_Temp>"
  Configuration_Check/6(MCU_Config_Parameter_No) -> Bus Creator/6  "MCU_Config_Param_No"
  Bus Selector/2 -> Temp_Check/2(Motor_Temp)  "<MCU_Temp>"

== system TBRe18_ECU_V7_AI/Data_Processing/Diagnostics/Shutdown_System_Diagnostics ==
  In1 : Inport
  Bus Creator : BusCreator  Inputs=1
  Constant : Constant  Value=false
  Terminator : Terminator
  Out1 : Outport
  wires:
  Bus Creator/1 -> Out1/1
  Constant/1 -> Bus Creator/1  "Shutdown_Error"
  In1/1 -> Terminator/1

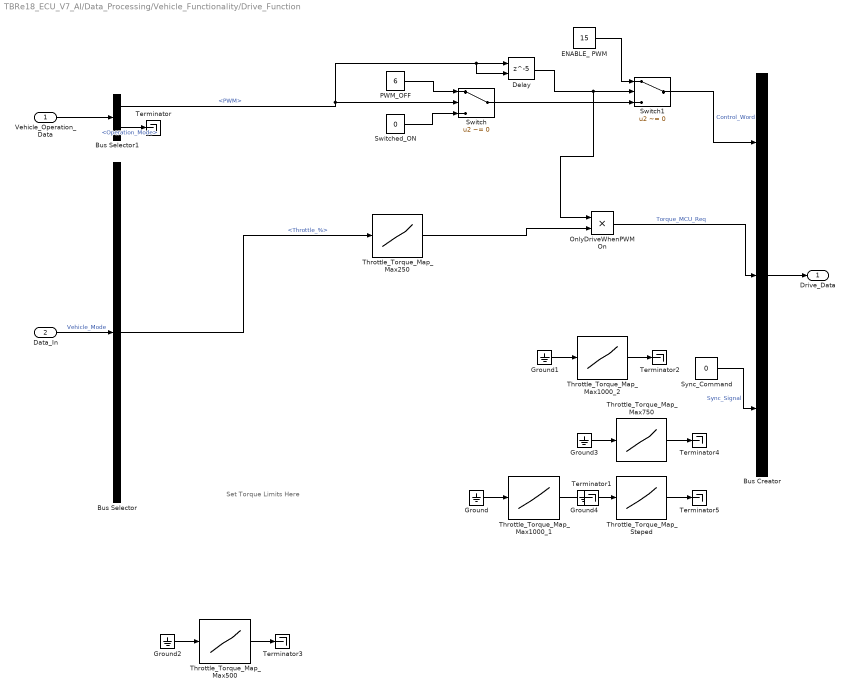
== system TBRe18_ECU_V7_AI/Data_Processing/Vehicle_Functionality/Drive_Function ==
  note: Set Torque Limits Here
  Vehicle_Operation_Data : Inport
  Data_In : Inport  Port=2
  Bus Creator : BusCreator  Inputs=3
  Bus Selector : BusSelector  OutputSignals=ECU_IO_Data.Pedal_Box_Data.Throttle_%
  Bus Selector1 : BusSelector  OutputSignals=PWM,Operation_Mode
  Delay : Delay  DelayLength=5  ExternalReset=Falling
      settings: InputPortMap=u0,r5
  ENABLE_ PWM : Constant  Value=15  OutDataTypeStr=uint16
  Ground{,1..4} (5 alike) : Ground
  OnlyDriveWhenPWMOn : Product  OutDataTypeStr=int16
  PWM_OFF : Constant  Value=6  OutDataTypeStr=uint16
  Switch : Switch  Criteria=u2 ~= 0  OutDataTypeStr=uint16
  Switch1 : Switch  Criteria=u2 ~= 0  OutDataTypeStr=uint16
  Switched_ON : Constant  Value=0  OutDataTypeStr=uint16
  "Sync_Command " : Constant  Value=0  OutDataTypeStr=uint8  SampleTime=-1
  Terminator{,1..5} (6 alike) : Terminator
  Throttle_Torque_Map_Max1000_1 : Lookup_n-D  NumberOfTableDimensions=1  BreakpointsForDimension1=[0,30,75,95,100]  Table=[0,100,650,800,1000]  ExtrapMethod=Clip  UseLastTableValue=on  InternalRulePriority=Speed  OutDataTypeStr=uint16  RndMeth=Simplest  InputSameDT=on
  Throttle_Torque_Map_Max1000_2 : Lookup_n-D  NumberOfTableDimensions=1  BreakpointsForDimension1=[0,30,75,95,100]  Table=[0,100,650,800,1000]  ExtrapMethod=Clip  UseLastTableValue=on  InternalRulePriority=Speed  OutDataTypeStr=uint16  RndMeth=Simplest  InputSameDT=on
  Throttle_Torque_Map_Max250 : Lookup_n-D  NumberOfTableDimensions=1  BreakpointsForDimension1=[0,30,75,100]  Table=[0,15,200,250]  ExtrapMethod=Clip  UseLastTableValue=on  InternalRulePriority=Speed  OutDataTypeStr=int16  RndMeth=Simplest  InputSameDT=on
  Throttle_Torque_Map_Max500 : Lookup_n-D  NumberOfTableDimensions=1  BreakpointsForDimension1=[0,30,75,100]  Table=[0,30,400,500]  ExtrapMethod=Clip  UseLastTableValue=on  InternalRulePriority=Speed  OutDataTypeStr=int16  RndMeth=Simplest  InputSameDT=on
  Throttle_Torque_Map_Max750 : Lookup_n-D  NumberOfTableDimensions=1  BreakpointsForDimension1=[0,30,75,100]  Table=[0,100,600,750]  ExtrapMethod=Clip  UseLastTableValue=on  InternalRulePriority=Speed  OutDataTypeStr=uint16  RndMeth=Simplest  InputSameDT=on
  Throttle_Torque_Map_Steped : Lookup_n-D  NumberOfTableDimensions=1  BreakpointsForDimension1=[0,20,40,60,70,90,100]  Table=[0,90,500,500,800,800,1000]  ExtrapMethod=Clip  UseLastTableValue=on  InternalRulePriority=Speed  OutDataTypeStr=uint16  RndMeth=Simplest  InputSameDT=on
  Drive_Data : Outport
  wires:
  "Sync_Command "/1 -> Bus Creator/3  "Sync_Signal"
  PWM_OFF/1 -> Switch/1
  Switched_ON/1 -> Switch/3
  Switch/1 -> Switch1/3
  ENABLE_ PWM/1 -> Switch1/1
  Delay/1 -> OnlyDriveWhenPWMOn/1, Switch1/2
  Switch1/1 -> Bus Creator/1  "Control_Word"
  Bus Creator/1 -> Drive_Data/1
  OnlyDriveWhenPWMOn/1 -> Bus Creator/2  "Torque_MCU_Req"
  Data_In/1 -> Bus Selector/1  "Vehicle_Mode"
  Vehicle_Operation_Data/1 -> Bus Selector1/1
  Bus Selector1/1 -> Delay/2, Delay/1, Switch/2  "<PWM>"
  Throttle_Torque_Map_Max250/1 -> OnlyDriveWhenPWMOn/2
  Bus Selector/1 -> Throttle_Torque_Map_Max250/1  "<Throttle_%>"
  Bus Selector1/2 -> Terminator/1  "<Operation_Mode>"
  Ground/1 -> Throttle_Torque_Map_Max1000_1/1
  Throttle_Torque_Map_Max1000_1/1 -> Terminator1/1
  Ground1/1 -> Throttle_Torque_Map_Max1000_2/1
  Throttle_Torque_Map_Max1000_2/1 -> Terminator2/1
  Ground2/1 -> Throttle_Torque_Map_Max500/1
  Throttle_Torque_Map_Max500/1 -> Terminator3/1
  Ground3/1 -> Throttle_Torque_Map_Max750/1
  Throttle_Torque_Map_Max750/1 -> Terminator4/1
  Ground4/1 -> Throttle_Torque_Map_Steped/1
  Throttle_Torque_Map_Steped/1 -> Terminator5/1

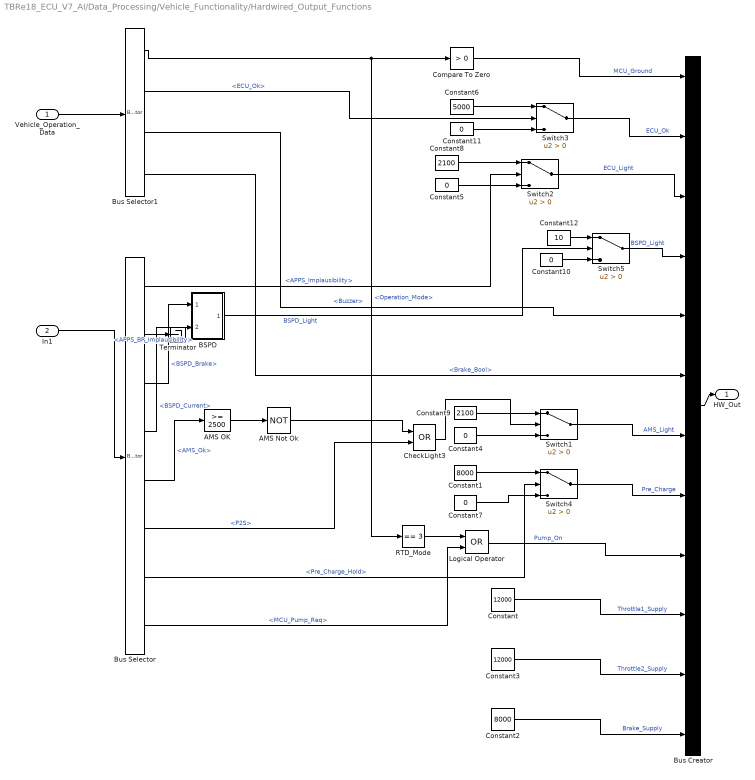
== system TBRe18_ECU_V7_AI/Data_Processing/Vehicle_Functionality/Hardwired_Output_Functions ==
  Vehicle_Operation_Data : Inport
  In1 : Inport  Port=2
  AMS Not Ok : Logic  Operator=NOT  AllPortsSameDT=off  OutDataTypeStr=boolean
  AMS OK : simulink/Logic and Bit Operations/Compare To Constant  relop=>=  const=2500  OutDataTypeStr=boolean
  BSPD : Subsystem
  Bus Creator : BusCreator  Inputs=12
  Bus Selector : BusSelector  OutputSignals=ECU_IO_Data.Pedal_Box_Data.APPS_Implausibility,ECU_IO_Data.Pedal_Box_Data.APPS_BP_Implausibility,Raw_Input_Data.Hardwired_Inputs.Pedal_Box_Data.BSPD_Brake,Raw_Input_Data.Hardwired_Inputs.Pedal_Box_Data.BSPD_Current,Raw_Input_Data.Hardwired_Inputs.AMS_Ok,Console_Data.P2S,BMS_Data.Pre_Charge_Hold,MCU_Data.MCU_Pump_Req
  Bus Selector1 : BusSelector  OutputSignals=Operation_Mode,ECU_Ok,Buzzer,Brake_Bool
  CheckLight3 : Logic  Operator=OR  AllPortsSameDT=off  OutDataTypeStr=boolean
  Compare To Zero : simulink/Logic and Bit Operations/Compare To Zero  relop=>  OutDataTypeStr=boolean
  Constant : Constant  Value=12000  OutDataTypeStr=uint16
  Constant1 : Constant  Value=8000  OutDataTypeStr=Inherit: Inherit via back propagation
  Constant{4..5,10..11} (4 alike) : Constant  Value=0  OutDataTypeStr=uint16
  Constant12 : Constant  Value=10  OutDataTypeStr=uint16
  Constant2 : Constant  Value=8000  OutDataTypeStr=uint16
  Constant3 : Constant  Value=12000  OutDataTypeStr=uint16
  Constant6 : Constant  Value=5000  OutDataTypeStr=uint16
  Constant7 : Constant  Value=0  OutDataTypeStr=Inherit: Inherit via back propagation
  Constant8 : Constant  Value=2100  OutDataTypeStr=uint16
  Constant9 : Constant  Value=2100  OutDataTypeStr=uint16
  Logical Operator : Logic  Operator=OR  AllPortsSameDT=off  OutDataTypeStr=boolean
  RTD_Mode : simulink/Logic and Bit Operations/Compare To Constant  relop===  const=3  OutDataTypeStr=boolean
  Switch1 : Switch  Criteria=u2 > Threshold  OutDataTypeStr=uint16
  Switch2 : Switch  Criteria=u2 > Threshold
  Switch3 : Switch  Criteria=u2 > Threshold
  Switch4 : Switch  Criteria=u2 > Threshold  OutDataTypeStr=uint16
  Switch5 : Switch  Criteria=u2 > Threshold
  Terminator : Terminator
  HW_Out : Outport
  wires:
  Constant/1 -> Bus Creator/10  "Throttle1_Supply"
  Bus Creator/1 -> HW_Out/1
  Constant2/1 -> Bus Creator/12  "Brake_Supply"
  Constant3/1 -> Bus Creator/11  "Throttle2_Supply"
  In1/1 -> Bus Selector/1
  Bus Selector/8 -> Logical Operator/2  "<MCU_Pump_Req>"
  Compare To Zero/1 -> Bus Creator/1  "MCU_Ground"
  Switch1/1 -> Bus Creator/7  "AMS_Light"
  Bus Selector/5 -> AMS OK/1  "<AMS_Ok>"
  Switch4/1 -> Bus Creator/8  "Pre_Charge"
  Switch3/1 -> Bus Creator/2  "ECU_Ok"
  Constant1/1 -> Switch4/1
  Bus Selector/7 -> Switch4/2  "<Pre_Charge_Hold>"
  Constant6/1 -> Switch3/1
  Constant7/1 -> Switch4/3
  Vehicle_Operation_Data/1 -> Bus Selector1/1
  Bus Selector1/1 -> Compare To Zero/1, RTD_Mode/1  "<Operation_Mode>"
  Bus Selector1/2 -> Switch3/2  "<ECU_Ok>"
  Constant4/1 -> Switch1/3
  Constant9/1 -> Switch1/1
  Constant11/1 -> Switch3/3
  Bus Selector/4 -> BSPD/2(In3)  "<BSPD_Current>"
  Bus Selector/3 -> BSPD/1(In1)  "<BSPD_Brake>"
  AMS OK/1 -> AMS Not Ok/1
  Bus Selector/6 -> CheckLight3/2  "<P2S>"
  CheckLight3/1 -> Switch1/2
  AMS Not Ok/1 -> CheckLight3/1
  Bus Selector1/4 -> Bus Creator/6  "<Brake_Bool>"
  Bus Selector1/3 -> Bus Creator/5  "<Buzzer>"
  BSPD/1(Out1) -> Switch5/2  "BSPD_Light"
  Bus Selector/1 -> Switch2/2  "<APPS_Implausibility>"
  RTD_Mode/1 -> Logical Operator/1
  Logical Operator/1 -> Bus Creator/9  "Pump_On"
  Switch2/1 -> Bus Creator/3  "ECU_Light"
  Constant5/1 -> Switch2/3
  Constant8/1 -> Switch2/1
  Switch5/1 -> Bus Creator/4  "BSPD_Light"
  Constant12/1 -> Switch5/1
  Constant10/1 -> Switch5/3
  Bus Selector/2 -> Terminator/1  "<APPS_BP_Implausibility>"

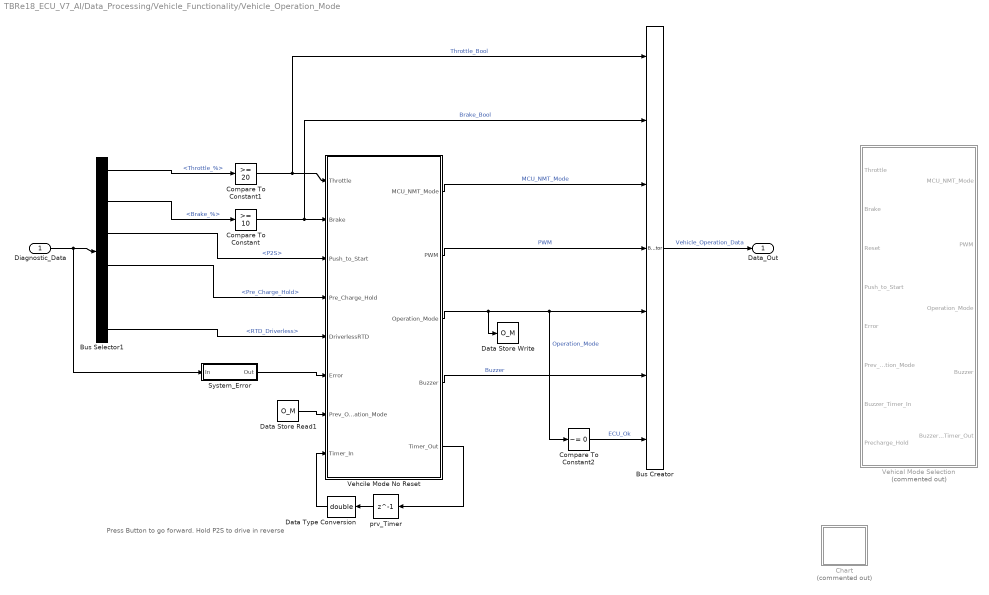
== system TBRe18_ECU_V7_AI/Data_Processing/Vehicle_Functionality/Vehicle_Operation_Mode ==
  note: Press Button to go forward. Hold P2S to drive in reverse
  Diagnostic_Data : Inport
  Bus Creator : BusCreator  Inputs=7
  Bus Selector1 : BusSelector  OutputSignals=ECU_IO_Data.Pedal_Box_Data.Throttle_%,ECU_IO_Data.Pedal_Box_Data.Brake_%,Console_Data.P2S,BMS_Data.Pre_Charge_Hold,Raw_Input_Data.Hardwired_Inputs.Console_Data.Push_to_Start,Raw_Input_Data.Hardwired_Inputs.RTD_Driverless
  Chart : Stateflow chart  Commented=on  TreatAsAtomicUnit=on
  Compare To Constant : simulink/Logic and Bit Operations/Compare To Constant  relop=>=  const=10  OutDataTypeStr=boolean
  Compare To Constant1 : simulink/Logic and Bit Operations/Compare To Constant  relop=>=  const=20  OutDataTypeStr=boolean
  Compare To Constant2 : simulink/Logic and Bit Operations/Compare To Constant  relop=~=  const=0  OutDataTypeStr=boolean
  Data Store Read1 : DataStoreRead  DataStoreName=O_M
  Data Store Write : DataStoreWrite  DataStoreName=O_M
  Data Type Conversion : DataTypeConversion  OutDataTypeStr=double
  System_Error : Subsystem
  Vehcile Mode No Reset : MATLAB Function  TreatAsAtomicUnit=on
  Vehical Mode Selection : MATLAB Function  Commented=on  TreatAsAtomicUnit=on
  prv_Timer : Delay  DelayLength=1  InitialCondition=0
  Data_Out : Outport
  wires:
  Bus Creator/1 -> Data_Out/1  "Vehicle_Operation_Data"
  Vehcile Mode No Reset/3(Operation_Mode) -> Data Store Write/1, Compare To Constant2/1, Bus Creator/5  "Operation_Mode"
  Vehcile Mode No Reset/1(MCU_NMT_Mode) -> Bus Creator/3  "MCU_NMT_Mode"
  Diagnostic_Data/1 -> Bus Selector1/1, System_Error/1(In)
  Bus Selector1/3 -> Vehcile Mode No Reset/3(Push_to_Start)  "<P2S>"
  Vehcile Mode No Reset/2(PWM) -> Bus Creator/4  "PWM"
  Compare To Constant1/1 -> Vehcile Mode No Reset/1(Throttle), Bus Creator/1  "Throttle_Bool"
  Compare To Constant/1 -> Bus Creator/2, Vehcile Mode No Reset/2(Brake)  "Brake_Bool"
  Vehcile Mode No Reset/5(Timer_Out) -> prv_Timer/1
  Vehcile Mode No Reset/4(Buzzer) -> Bus Creator/6  "Buzzer"
  Bus Selector1/1 -> Compare To Constant1/1  "<Throttle_%>"
  Bus Selector1/2 -> Compare To Constant/1  "<Brake_%>"
  Compare To Constant2/1 -> Bus Creator/7  "ECU_Ok"
  System_Error/1(Out) -> Vehcile Mode No Reset/6(Error)
  Bus Selector1/4 -> Vehcile Mode No Reset/4(Pre_Charge_Hold)  "<Pre_Charge_Hold>"
  Data Store Read1/1 -> Vehcile Mode No Reset/7(Prev_Operation_Mode)
  prv_Timer/1 -> Data Type Conversion/1
  Data Type Conversion/1 -> Vehcile Mode No Reset/8(Timer_In)
  Bus Selector1/6 -> Vehcile Mode No Reset/5(DriverlessRTD)  "<RTD_Driverless>"

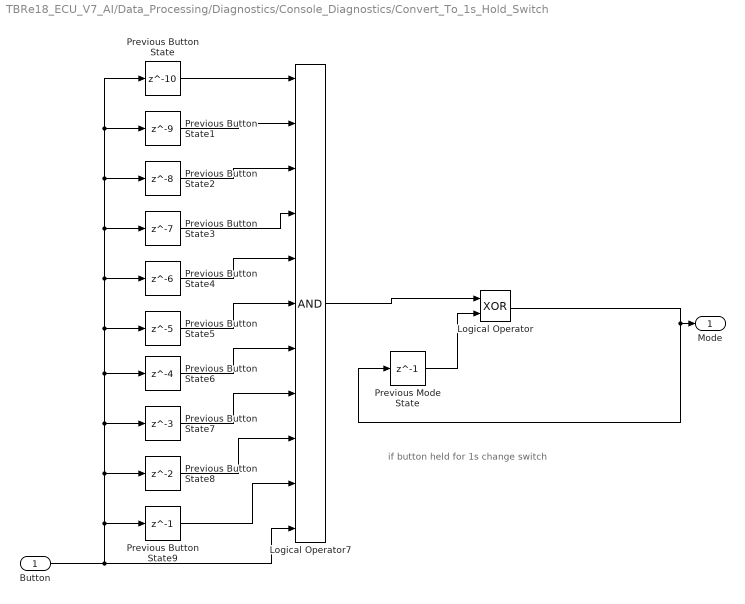
== system TBRe18_ECU_V7_AI/Data_Processing/Diagnostics/Console_Diagnostics/Convert_To_1s_Hold_Switch ==
  note: if button held for 1s change switch
  Button : Inport
  Logical Operator : Logic  Operator=XOR  AllPortsSameDT=off  OutDataTypeStr=boolean
  Logical Operator7 : Logic  Inputs=11  AllPortsSameDT=off  OutDataTypeStr=boolean
  Previous Button State : Delay  DelayLength=10  InitialCondition=initPos
  Previous Button State1 : Delay  DelayLength=9  InitialCondition=initPos
  Previous Button State2 : Delay  DelayLength=8  InitialCondition=initPos
  Previous Button State3 : Delay  DelayLength=7  InitialCondition=initPos
  Previous Button State4 : Delay  DelayLength=6  InitialCondition=initPos
  Previous Button State5 : Delay  DelayLength=5  InitialCondition=initPos
  Previous Button State6 : Delay  DelayLength=4  InitialCondition=initPos
  Previous Button State7 : Delay  DelayLength=3  InitialCondition=initPos
  Previous Button State8 : Delay  InitialCondition=initPos
  Previous Button State9 : Delay  DelayLength=1  InitialCondition=initPos
  Previous Mode State : Delay  DelayLength=1  InitialCondition=false
  Mode : Outport
  wires:
  Logical Operator/1 -> Previous Mode State/1, Mode/1
  Previous Button State/1 -> Logical Operator7/1
  Previous Button State1/1 -> Logical Operator7/2
  Previous Button State2/1 -> Logical Operator7/3
  Previous Button State3/1 -> Logical Operator7/4
  Previous Button State4/1 -> Logical Operator7/5
  Previous Button State5/1 -> Logical Operator7/6
  Previous Button State6/1 -> Logical Operator7/7
  Previous Button State7/1 -> Logical Operator7/8
  Previous Button State8/1 -> Logical Operator7/9
  Previous Button State9/1 -> Logical Operator7/10
  Button/1 -> Previous Button State9/1, Previous Button State8/1, Previous Button State7/1, Previous Button State6/1, Previous Button State5/1, Previous Button State4/1, Previous Button State3/1, Previous Button State2/1, Previous Button State1/1, Previous Button State/1, Logical Operator7/11
  Logical Operator7/1 -> Logical Operator/1
  Previous Mode State/1 -> Logical Operator/2

== system TBRe18_ECU_V7_AI/Data_Processing/Diagnostics/Console_Diagnostics/Convert_To_Switch ==
  note: Calculated from Boolean Logic:
      |
      | Changes Mode on a rasing edge
      |
      | if((button == true) && (prvbutton == false))
      |     Mode = ~prvMode;
      | else
      |     Mode = prvMode;
      | end
  Button : Inport
  Logical Operator : Logic  AllPortsSameDT=off  OutDataTypeStr=boolean
  Logical Operator1 : Logic  AllPortsSameDT=off  OutDataTypeStr=boolean
  Logical Operator2 : Logic  Inputs=3  AllPortsSameDT=off  OutDataTypeStr=boolean
  Logical Operator3 : Logic  Operator=OR  Inputs=3  AllPortsSameDT=off  OutDataTypeStr=boolean
  Logical Operator4 : Logic  Operator=NOT  AllPortsSameDT=off  OutDataTypeStr=boolean
  Logical Operator5 : Logic  Operator=NOT  AllPortsSameDT=off  OutDataTypeStr=boolean
  Logical Operator6 : Logic  Operator=NOT  AllPortsSameDT=off  OutDataTypeStr=boolean
  Previous Button State : Delay  DelayLength=1  InitialCondition=false
  Previous Mode State : Delay  DelayLength=1  InitialCondition=initPos
  Mode : Outport
  wires:
  Button/1 -> Logical Operator5/1, Previous Button State/1, Logical Operator2/2
  Previous Mode State/1 -> Logical Operator1/2, Logical Operator6/1, Logical Operator/2
  Logical Operator5/1 -> Logical Operator/1
  Previous Button State/1 -> Logical Operator1/1, Logical Operator4/1
  Logical Operator4/1 -> Logical Operator2/1
  Logical Operator/1 -> Logical Operator3/1
  Logical Operator3/1 -> Mode/1, Previous Mode State/1
  Logical Operator6/1 -> Logical Operator2/3
  Logical Operator1/1 -> Logical Operator3/2
  Logical Operator2/1 -> Logical Operator3/3

== system TBRe18_ECU_V7_AI/Data_Processing/Diagnostics/Console_Diagnostics/Convert_To_Switch_Simplified ==
  note: Calculated from Boolean Logic:
      |
      | Changes Mode on a rasing edge
      |
      | if((button == true) && (prvbutton == false))
      |     Mode = ~prvMode;
      | else
      |     Mode = prvMode;
      | end
  note: P2S only acts on down press
  Button : Inport
  Logical Operator7 : Logic  Operator=NOT  AllPortsSameDT=off  OutDataTypeStr=boolean
  Logical Operator8 : Logic  AllPortsSameDT=off  OutDataTypeStr=boolean
  Logical Operator9 : Logic  Operator=XOR  AllPortsSameDT=off  OutDataTypeStr=boolean
  Previous Mode State : Delay  DelayLength=1  InitialCondition=initPos
  prvP2S : Delay  DelayLength=1  InitialCondition=0
  Mode : Outport
  wires:
  Previous Mode State/1 -> Logical Operator9/2
  Logical Operator7/1 -> Logical Operator8/2
  prvP2S/1 -> Logical Operator7/1
  Logical Operator8/1 -> Logical Operator9/1  "P2S"
  Button/1 -> Logical Operator8/1, prvP2S/1
  Logical Operator9/1 -> Previous Mode State/1, Mode/1

== system TBRe18_ECU_V7_AI/Data_Processing/Diagnostics/ECU_I//0s_Diagnostics/AIR ==
  note: AIR open = 0V
      | AIR closed = 5V
  note: Need additional info on the AIR
  In1 : Inport
  Bus Creator : BusCreator  Inputs=1
  Bus Selector : BusSelector  OutputSignals=AIR
  Compare To Zero : simulink/Logic and Bit Operations/Compare To Zero  relop===  OutDataTypeStr=boolean
  Out1 : Outport
  wires:
  Bus Creator/1 -> Out1/1
  In1/1 -> Bus Selector/1
  Bus Selector/1 -> Compare To Zero/1  "<AIR>"
  Compare To Zero/1 -> Bus Creator/1  "AIR_Error"

== system TBRe18_ECU_V7_AI/Data_Processing/Diagnostics/ECU_I//0s_Diagnostics/IMD ==
  note: Need additional info on the IMD about level of frequency (2018)
      | Spec on x Drive:
      |
      | This works so not changed (2019)
  In1 : Inport
  Bus Creator : BusCreator  Inputs=1
  Constant : Constant  Value=false
  Terminator : Terminator
  Out1 : Outport
  wires:
  Bus Creator/1 -> Out1/1
  Constant/1 -> Bus Creator/1  "ECU_IMD_Error"
  In1/1 -> Terminator/1
